simulink model "ACCLogic_Test"  (Simulink 7.8)
settings: Solver=ode3  StartTime=0.0  StopTime=35  FixedStep=TIMESTEP  RelTol=1e-3
InitFcn:
  | ACCLogic_TestCase1
StopFcn:
  | ACCLogic_plot
values from neighbouring files (symbols this model uses):
  Car1_start_s = 140    [ACCLogic_TestCase1.m]    (also in ACCLogic_TestCase2.m = 30)
  Car1_us = 0    [ACCLogic_TestCase1.m]    (also in ACCLogic_TestCase2.m)
  Car2_start_s = 47    [ACCLogic_TestCase1.m]    (also in ACCLogic_TestCase2.m)
  Car2_us = 1    [ACCLogic_TestCase1.m]    (also in ACCLogic_TestCase2.m)
  Car3_start_s = 25    [ACCLogic_TestCase1.m]    (also in ACCLogic_TestCase2.m)
  Car3_us = 0.25    [ACCLogic_TestCase1.m]    (also in ACCLogic_TestCase2.m)
  Car4_start_s = 95    [ACCLogic_TestCase1.m]    (also in ACCLogic_TestCase2.m = 35)
  Car4_us = 0.5    [ACCLogic_TestCase1.m]    (also in ACCLogic_TestCase2.m)
  Car5_start_s = 141    [ACCLogic_TestCase1.m]    (also in ACCLogic_TestCase2.m = 75)
  Car5_us = 0    [ACCLogic_TestCase1.m]    (also in ACCLogic_TestCase2.m)
  H = 10    [ACCLogic_TestCase1.m]    (also in ACCLogic_TestCase2.m)
  ManEnt1 = 10    [ACCLogic_TestCase1.m]    (also in ACCLogic_TestCase2.m)
  ManEnt2 = 15    [ACCLogic_TestCase1.m]    (also in ACCLogic_TestCase2.m)
  ManEnt3 = 20    [ACCLogic_TestCase1.m]    (also in ACCLogic_TestCase2.m)
  ManEnt4 = 25    [ACCLogic_TestCase1.m]    (also in ACCLogic_TestCase2.m)
  MyCarMan_us = 6    [ACCLogic_TestCase1.m]    (also in ACCLogic_TestCase2.m)
  MyCarVel_us = 3    [ACCLogic_TestCase1.m]    (also in ACCLogic_TestCase2.m)
  TIMESTEP = 0.01    [ACCLogic_TestCase1.m]    (also in ACCLogic_TestCase2.m)
libraries: simulink x5
settings Model: Creator=jmapatel  LastModifiedBy=cjzhang
settings DebuggingCC: FrameProcessingCompatibilityMsg=error
settings CodeAppCC: CustomSymbolStrType=$N$R$M_T
settings GRTTargetCC: TargetFunctionLibrary=NOT IN USE  CPPClassGenCompliant=on

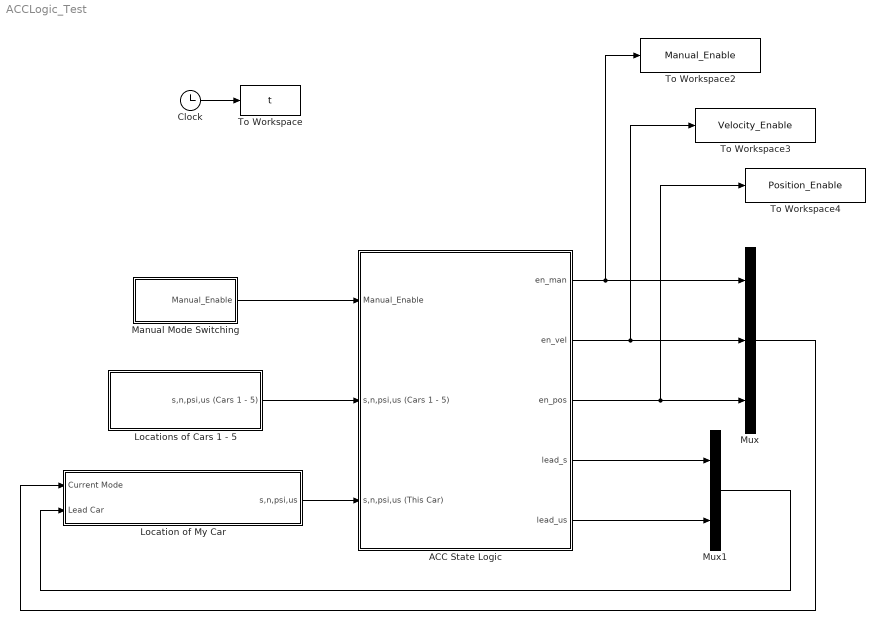
== system ACCLogic_Test ==
  ACC State Logic : Subsystem
  Clock : Clock
  Location of My Car : Subsystem
  Locations of Cars 1 - 5 : Subsystem
  Manual Mode Switching : Subsystem
  Mux : Mux  Inputs=3
  Mux1 : Mux  Inputs=2
  To Workspace : ToWorkspace  VariableName=t  SampleTime=-1  SaveFormat=Array
  To Workspace2 : ToWorkspace  VariableName=Manual_Enable  SampleTime=-1  SaveFormat=Array
  To Workspace3 : ToWorkspace  VariableName=Velocity_Enable  SampleTime=-1  SaveFormat=Array
  To Workspace4 : ToWorkspace  VariableName=Position_Enable  SampleTime=-1  SaveFormat=Array
  wires:
  Clock/1 -> To Workspace/1
  Manual Mode Switching/1(Manual_Enable) -> ACC State Logic/1(Manual_Enable)
  Locations of Cars 1 - 5/1(s,n,psi,us (Cars 1 - 5)) -> ACC State Logic/2(s,n,psi,us (Cars 1 - 5))
  Location of My Car/1(s,n,psi,us) -> ACC State Logic/3(s,n,psi,us (This Car))
  ACC State Logic/1(en_man) -> Mux/1, To Workspace2/1
  ACC State Logic/2(en_vel) -> Mux/2, To Workspace3/1
  ACC State Logic/3(en_pos) -> Mux/3, To Workspace4/1
  ACC State Logic/4(lead_s) -> Mux1/1
  ACC State Logic/5(lead_us) -> Mux1/2
  Mux/1 -> Location of My Car/1(Current Mode)
  Mux1/1 -> Location of My Car/2(Lead Car)

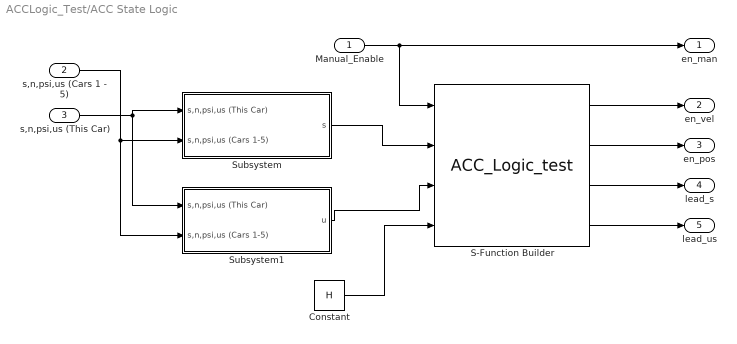
== system ACCLogic_Test/ACC State Logic ==
  Manual_Enable : Inport
  s,n,psi,us (Cars 1 - 5) : Inport  Port=2
  s,n,psi,us (This Car) : Inport  Port=3
  Constant : Constant  Value=H  OutDataTypeStr=single
  S-Function Builder : S-Function  InitFcn=try, set_param(gcb,'FunctionName','ACC_Logic_test'), end  FunctionName=ACC_Logic_test  SFunctionModules=ACC_Logic_test_wrapper  WizardData=DataTag0  EnableBusSupport=off
      mask init:
      | val = [[.9  0.75 0.75 1 1 .9 .9 1]',[1 1 0.75 0.75 .9 .9 1 .9]'];try , sys = get_param(gcb,'SfunBuilderFcnName');if isempty(sys), sys = get_param(gcb,'FunctionName'); end,catch, sys = get_param(gcb,'FunctionName'); end
      settings: CopyFcn=set_param(gcbh,'LinkStatus','none')  PreSaveFcn=try, set_param(gcb,'FunctionName','ACC_Logic_test'), end  OpenFcn=sfunctionwizard(gcbh)
      mask Display: plot(val(:,1),val(:,2)),disp(sys), port_label('input',1,'en_man'), port_label('input',2,'s'), port_label('input',3,'u'), port_label('input',4,'H'), port_label('output',1,'en_vel'), port_label('output',2,'en_pos'), port_label('output',3,'lead_s'), port_label('output',4,'lead_us')
  Subsystem : Subsystem
  Subsystem1 : Subsystem
  en_man : Outport
  en_vel : Outport  Port=2
  en_pos : Outport  Port=3
  lead_s : Outport  Port=4
  lead_us : Outport  Port=5
  wires:
  s,n,psi,us (This Car)/1 -> Subsystem/1(s,n,psi,us (This Car)), Subsystem1/1(s,n,psi,us (This Car))
  s,n,psi,us (Cars 1 - 5)/1 -> Subsystem1/2(s,n,psi,us (Cars 1-5)), Subsystem/2(s,n,psi,us (Cars 1-5))
  Manual_Enable/1 -> en_man/1, S-Function Builder/1
  Subsystem/1(s) -> S-Function Builder/2
  Subsystem1/1(u) -> S-Function Builder/3
  S-Function Builder/1 -> en_vel/1
  S-Function Builder/2 -> en_pos/1
  S-Function Builder/4 -> lead_us/1
  S-Function Builder/3 -> lead_s/1
  Constant/1 -> S-Function Builder/4

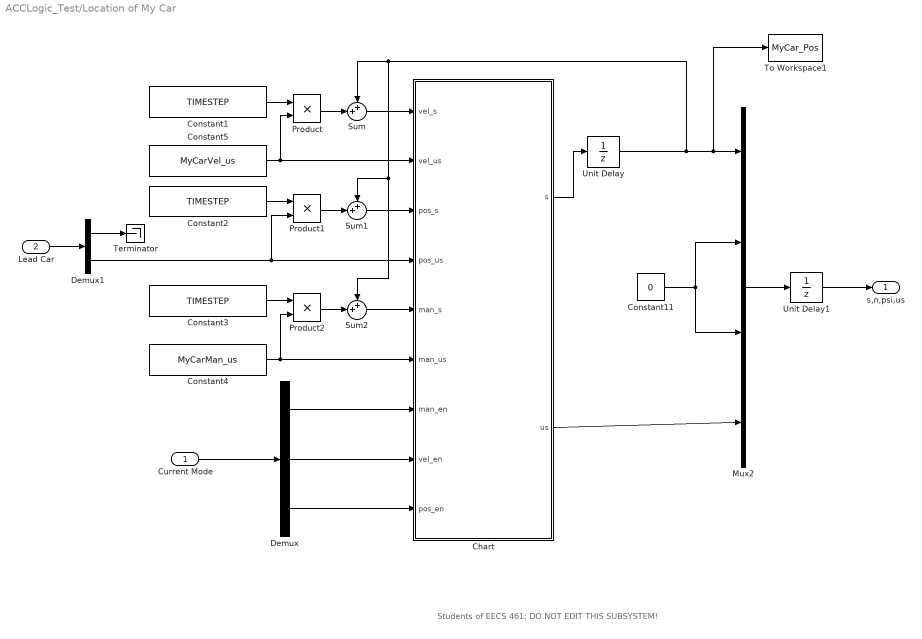
== system ACCLogic_Test/Location of My Car ==
  note: Students of EECS 461: DO NOT EDIT THIS SUBSYSTEM!
  Current Mode : Inport
  Lead Car : Inport  Port=2
  Chart : Stateflow chart  TreatAsAtomicUnit=on
  Constant1 : Constant  Value=TIMESTEP  OutDataTypeStr=single
  Constant11 : Constant  Value=0  OutDataTypeStr=single
  Constant2 : Constant  Value=TIMESTEP  OutDataTypeStr=single
  Constant3 : Constant  Value=TIMESTEP  OutDataTypeStr=single
  Constant4 : Constant  Value=MyCarMan_us  OutDataTypeStr=single
  Constant5 : Constant  Value=MyCarVel_us  OutDataTypeStr=single
  Demux : Demux  Outputs=3
  Demux1 : Demux  Outputs=2
  Mux2 : Mux
  Product : Product  RndMeth=Zero
  Product1 : Product  RndMeth=Zero
  Product2 : Product  RndMeth=Zero
  Sum : Sum  Inputs=++|
  Sum1 : Sum  Inputs=++|
  Sum2 : Sum  Inputs=++|
  Terminator : Terminator
  To Workspace1 : ToWorkspace  VariableName=MyCar_Pos  SampleTime=-1  SaveFormat=Array
  Unit Delay : UnitDelay  SampleTime=-1
  Unit Delay1 : UnitDelay  SampleTime=-1
  s,n,psi,us : Outport
  wires:
  Chart/2(us) -> Mux2/4
  Demux/1 -> Chart/7(man_en)
  Demux/2 -> Chart/8(vel_en)
  Demux/3 -> Chart/9(pos_en)
  Sum/1 -> Chart/1(vel_s)
  Product/1 -> Sum/2
  Constant1/1 -> Product/1
  Product1/1 -> Sum1/2
  Constant2/1 -> Product1/1
  Sum1/1 -> Chart/3(pos_s)
  Sum2/1 -> Chart/5(man_s)
  Product2/1 -> Sum2/2
  Constant3/1 -> Product2/1
  Chart/1(s) -> Unit Delay/1
  Unit Delay/1 -> Mux2/1, To Workspace1/1, Sum/1, Sum1/1, Sum2/1
  Mux2/1 -> Unit Delay1/1
  Unit Delay1/1 -> s,n,psi,us/1
  Current Mode/1 -> Demux/1
  Constant4/1 -> Chart/6(man_us), Product2/2
  Constant5/1 -> Chart/2(vel_us), Product/2
  Constant11/1 -> Mux2/2, Mux2/3
  Lead Car/1 -> Demux1/1
  Demux1/1 -> Terminator/1
  Demux1/2 -> Chart/4(pos_us), Product1/2

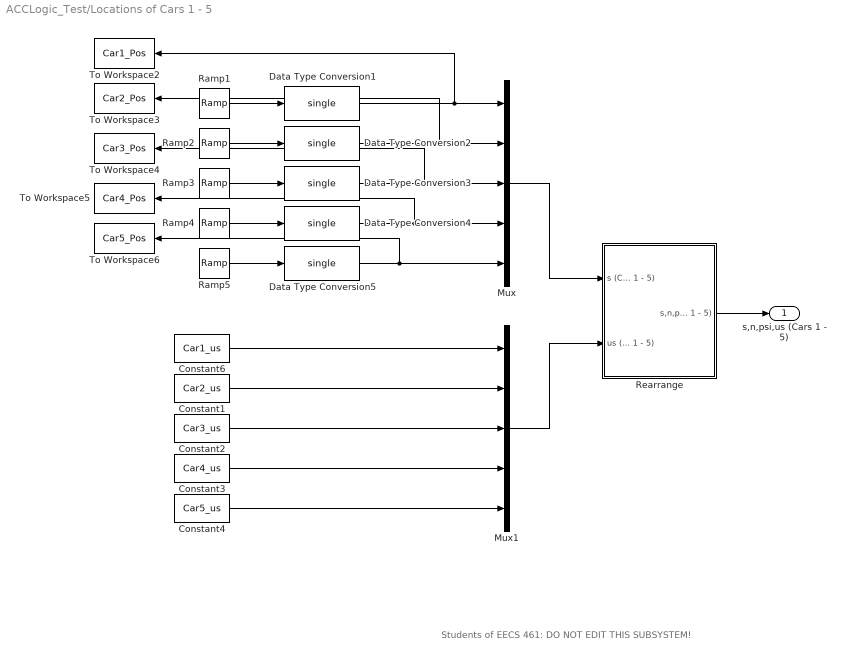
== system ACCLogic_Test/Locations of Cars 1 - 5 ==
  note: Students of EECS 461: DO NOT EDIT THIS SUBSYSTEM!
  Constant1 : Constant  Value=Car2_us  OutDataTypeStr=single
  Constant2 : Constant  Value=Car3_us  OutDataTypeStr=single
  Constant3 : Constant  Value=Car4_us  OutDataTypeStr=single
  Constant4 : Constant  Value=Car5_us  OutDataTypeStr=single
  Constant6 : Constant  Value=Car1_us  OutDataTypeStr=single
  Data Type Conversion{1..5} (5 alike) : DataTypeConversion  OutDataTypeStr=single
  Mux : Mux  Inputs=5
  Mux1 : Mux  Inputs=5
  Ramp1 : simulink/Sources/Ramp  slope=Car1_us  start=0  X0=Car1_start_s
  Ramp2 : simulink/Sources/Ramp  slope=Car2_us  start=0  X0=Car2_start_s
  Ramp3 : simulink/Sources/Ramp  slope=Car3_us  start=0  X0=Car3_start_s
  Ramp4 : simulink/Sources/Ramp  slope=Car4_us  start=0  X0=Car4_start_s
  Ramp5 : simulink/Sources/Ramp  slope=Car5_us  start=0  X0=Car5_start_s
  Rearrange : Subsystem
  To Workspace2 : ToWorkspace  VariableName=Car1_Pos  SampleTime=-1  SaveFormat=Array
  To Workspace3 : ToWorkspace  VariableName=Car2_Pos  SampleTime=-1  SaveFormat=Array
  To Workspace4 : ToWorkspace  VariableName=Car3_Pos  SampleTime=-1  SaveFormat=Array
  To Workspace5 : ToWorkspace  VariableName=Car4_Pos  SampleTime=-1  SaveFormat=Array
  To Workspace6 : ToWorkspace  VariableName=Car5_Pos  SampleTime=-1  SaveFormat=Array
  s,n,psi,us (Cars 1 - 5) : Outport
  wires:
  Constant6/1 -> Mux1/1
  Constant1/1 -> Mux1/2
  Constant2/1 -> Mux1/3
  Constant3/1 -> Mux1/4
  Constant4/1 -> Mux1/5
  Mux/1 -> Rearrange/1(s (Cars 1 - 5))
  Mux1/1 -> Rearrange/2(us (Cars 1 - 5))
  Ramp1/1 -> Data Type Conversion1/1
  Data Type Conversion1/1 -> Mux/1, To Workspace2/1
  Ramp2/1 -> Data Type Conversion2/1
  Data Type Conversion2/1 -> Mux/2, To Workspace3/1
  Ramp3/1 -> Data Type Conversion3/1
  Data Type Conversion3/1 -> Mux/3, To Workspace4/1
  Ramp4/1 -> Data Type Conversion4/1
  Data Type Conversion4/1 -> Mux/4, To Workspace5/1
  Ramp5/1 -> Data Type Conversion5/1
  Data Type Conversion5/1 -> Mux/5, To Workspace6/1
  Rearrange/1(s,n,psi,us (Cars 1 - 5)) -> s,n,psi,us (Cars 1 - 5)/1

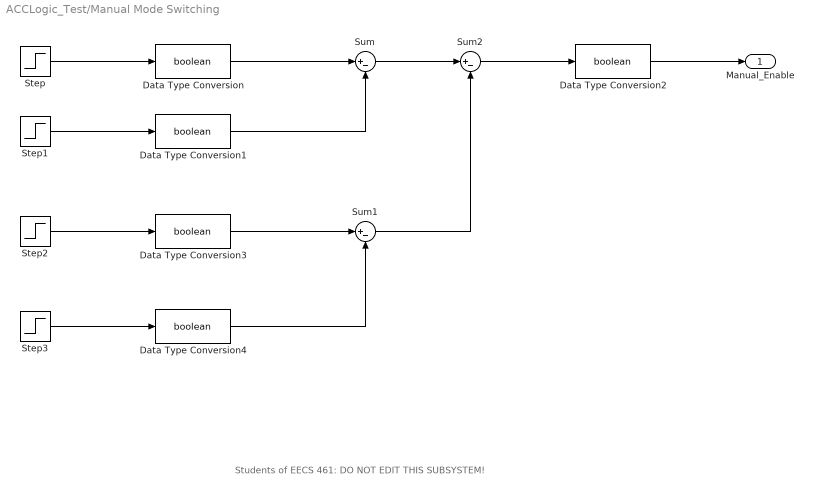
== system ACCLogic_Test/Manual Mode Switching ==
  note: Students of EECS 461: DO NOT EDIT THIS SUBSYSTEM!
  Data Type Conversion{,1..4} (5 alike) : DataTypeConversion  OutDataTypeStr=boolean
  Step : Step  Time=ManEnt1  SampleTime=0
  Step1 : Step  Time=ManEnt2  SampleTime=0
  Step2 : Step  Time=ManEnt3  SampleTime=0
  Step3 : Step  Time=ManEnt4  SampleTime=0
  Sum : Sum  Inputs=|+-
  Sum1 : Sum  Inputs=|+-
  Sum2 : Sum  Inputs=|+-
  Manual_Enable : Outport
  wires:
  Step/1 -> Data Type Conversion/1
  Step1/1 -> Data Type Conversion1/1
  Data Type Conversion/1 -> Sum/1
  Data Type Conversion1/1 -> Sum/2
  Data Type Conversion2/1 -> Manual_Enable/1
  Step2/1 -> Data Type Conversion3/1
  Step3/1 -> Data Type Conversion4/1
  Data Type Conversion3/1 -> Sum1/1
  Data Type Conversion4/1 -> Sum1/2
  Sum/1 -> Sum2/1
  Sum1/1 -> Sum2/2
  Sum2/1 -> Data Type Conversion2/1

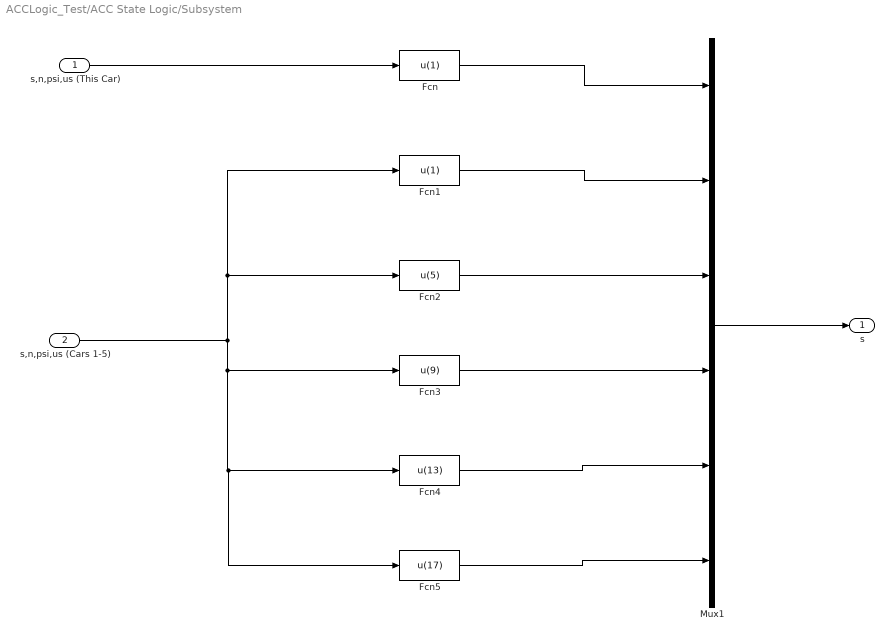
== system ACCLogic_Test/ACC State Logic/Subsystem ==
  s,n,psi,us (This Car) : Inport
  s,n,psi,us (Cars 1-5) : Inport  Port=2
  Fcn : Fcn  Expr=u(1)
  Fcn1 : Fcn  Expr=u(1)
  Fcn2 : Fcn  Expr=u(5)
  Fcn3 : Fcn  Expr=u(9)
  Fcn4 : Fcn  Expr=u(13)
  Fcn5 : Fcn  Expr=u(17)
  Mux1 : Mux  Inputs=6
  s : Outport
  wires:
  Fcn/1 -> Mux1/1
  Fcn4/1 -> Mux1/5
  Fcn3/1 -> Mux1/4
  Mux1/1 -> s/1
  Fcn5/1 -> Mux1/6
  Fcn2/1 -> Mux1/3
  Fcn1/1 -> Mux1/2
  s,n,psi,us (Cars 1-5)/1 -> Fcn3/1, Fcn5/1, Fcn4/1, Fcn2/1, Fcn1/1
  s,n,psi,us (This Car)/1 -> Fcn/1

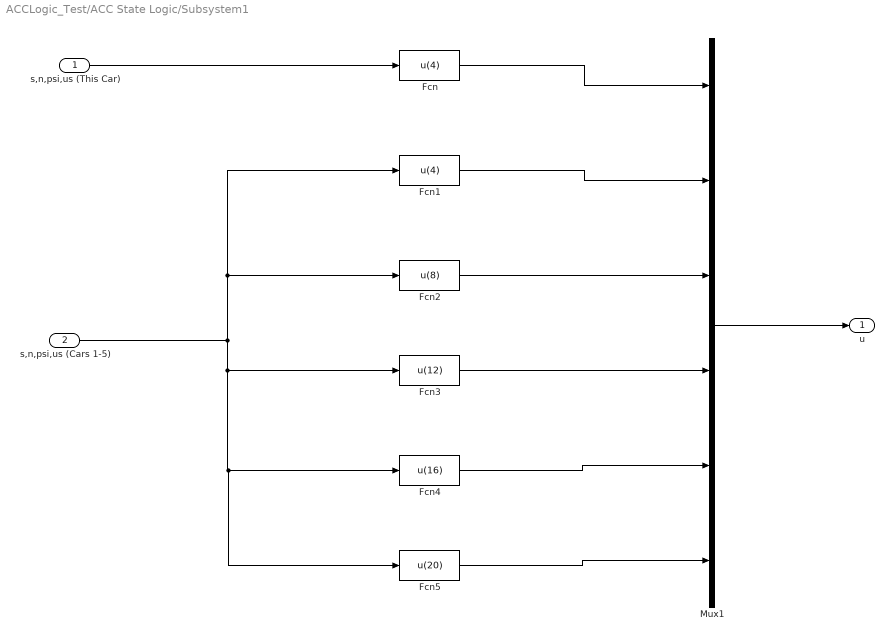
== system ACCLogic_Test/ACC State Logic/Subsystem1 ==
  s,n,psi,us (This Car) : Inport
  s,n,psi,us (Cars 1-5) : Inport  Port=2
  Fcn : Fcn  Expr=u(4)
  Fcn1 : Fcn  Expr=u(4)
  Fcn2 : Fcn  Expr=u(8)
  Fcn3 : Fcn  Expr=u(12)
  Fcn4 : Fcn  Expr=u(16)
  Fcn5 : Fcn  Expr=u(20)
  Mux1 : Mux  Inputs=6
  u : Outport
  wires:
  Fcn/1 -> Mux1/1
  Fcn4/1 -> Mux1/5
  Fcn3/1 -> Mux1/4
  Mux1/1 -> u/1
  Fcn5/1 -> Mux1/6
  Fcn2/1 -> Mux1/3
  Fcn1/1 -> Mux1/2
  s,n,psi,us (Cars 1-5)/1 -> Fcn3/1, Fcn5/1, Fcn4/1, Fcn2/1, Fcn1/1
  s,n,psi,us (This Car)/1 -> Fcn/1

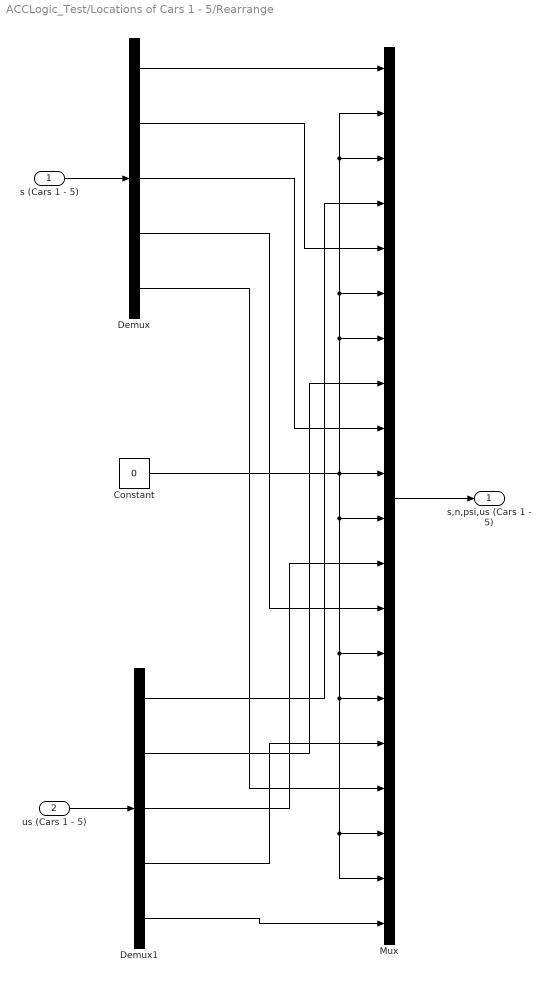
== system ACCLogic_Test/Locations of Cars 1 - 5/Rearrange ==
  s (Cars 1 - 5) : Inport
  us (Cars 1 - 5) : Inport  Port=2
  Constant : Constant  Value=0  OutDataTypeStr=single
  Demux : Demux  Outputs=5
  Demux1 : Demux  Outputs=5
  Mux : Mux  Inputs=20
  s,n,psi,us (Cars 1 - 5) : Outport
  wires:
  us (Cars 1 - 5)/1 -> Demux1/1
  s (Cars 1 - 5)/1 -> Demux/1
  Demux/1 -> Mux/1
  Constant/1 -> Mux/2, Mux/3, Mux/6, Mux/7, Mux/10, Mux/11, Mux/19, Mux/18, Mux/15, Mux/14
  Demux1/1 -> Mux/4
  Demux/2 -> Mux/5
  Demux1/2 -> Mux/8
  Demux/3 -> Mux/9
  Demux1/3 -> Mux/12
  Demux/4 -> Mux/13
  Demux1/4 -> Mux/16
  Demux/5 -> Mux/17
  Demux1/5 -> Mux/20
  Mux/1 -> s,n,psi,us (Cars 1 - 5)/1

== stateflow chart Location of My Car/Chart ==
  state vel_ctrl
    during:s = vel_s
    during:us = vel_us
  state pos_ctrl
    during:s = pos_s
    during:us = pos_us
  state man_ctrl
    during:s = man_s
    during:us = man_us
  (default) -> vel_ctrl
  vel_ctrl -> pos_ctrl [order 1] : [(pos_en==1)&(vel_en==0)&(man_en==0)]
  pos_ctrl -> vel_ctrl [order 1] : [(pos_en == 0)&(vel_en == 1)&(man_en == 0)]
  vel_ctrl -> man_ctrl [order 2] : [(pos_en == 0)&(vel_en == 0)&(man_en == 1)]
  man_ctrl -> vel_ctrl [order 2] : [(pos_en == 0)&(vel_en == 1)&(man_en == 0)]
  pos_ctrl -> man_ctrl [order 2] : [(pos_en == 0)&(vel_en == 0)&(man_en == 1)]
  man_ctrl -> pos_ctrl [order 1] : [(pos_en == 1)&(vel_en == 0)&(man_en == 0)]
  data: vel_s input single; vel_us input single; pos_s input single; pos_us input single; man_s input single; man_us input single; man_en input boolean; vel_en input boolean; pos_en input boolean; s output single; us output single
